simulink model "TiltCopter_Simulator"  (R2015a)
settings: Solver=ode45  StartTime=0.0  StopTime=10.0  RelTol=1e-3
values from neighbouring files (symbols this model uses):
  b = 0.55/2    (= 0.275)    [TiltCopter_Parameters.m]
  B0 = 1.399e04    (= 13990)    [TiltCopter_Parameters.m]
  B1 = 1150    [TiltCopter_Parameters.m]
  B2 = 37.46    [TiltCopter_Parameters.m]
  B3 = 1    [TiltCopter_Parameters.m]
  dLMN = [dLdp  0    0 ... (first row only)    [TiltCopter_Parameters.m]
  Fx = 0.5    [Main_tiltCopter.m]
  Fy = 0    [Main_tiltCopter.m]
  g = 9.81    [TiltCopter_Parameters.m]
  In = diag([Ixx Iyy Izz])    [TiltCopter_Parameters.m]
  InInv = In\eye(3)    [TiltCopter_Parameters.m]
  Kq = Cq*ro*A*R^3    (= 2.88925724261e-07)    [TiltCopter_Parameters.m]
  Kt = Ct*ro*A*R^2    (= 2.46191978476e-05)    [TiltCopter_Parameters.m]
  L = 0    [Main_tiltCopter.m]
  M = 0    [Main_tiltCopter.m]
  m = 1.478    [TiltCopter_Parameters.m]
  m_servo = p(1)    [TiltCopter_Parameters.m]
  Mb = diag([m m m])    [TiltCopter_Parameters.m]
  MbInv = Mb\eye(3)    [TiltCopter_Parameters.m]
  N = 0    [Main_tiltCopter.m]
  omega_hover = OMEhov    [TiltCopter_Parameters.m]
  q_servo = p(2)    [TiltCopter_Parameters.m]
  ServoMotor_Gain = 1.409e04    (= 14090)    [TiltCopter_Parameters.m]
  T = -20    [Main_tiltCopter.m]
  tau = 0.055257    [TiltCopter_Parameters.m]
  x1 = [m q]    [TiltCopter_Parameters.m]
libraries: aerolibutil x2
settings Model: Creator=Claudio  LastModifiedBy=Claudio

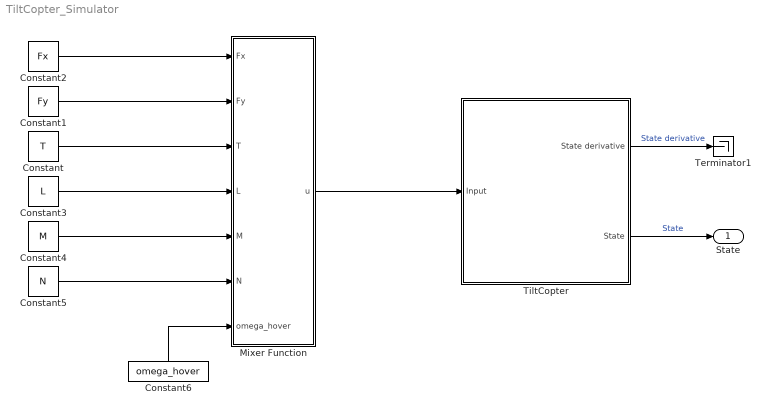
== system TiltCopter_Simulator ==
  Constant : Constant  Value=T
  Constant1 : Constant  Value=Fy
  Constant2 : Constant  Value=Fx
  Constant3 : Constant  Value=L
  Constant4 : Constant  Value=M
  Constant5 : Constant  Value=N
  Constant6 : Constant  Value=omega_hover
  Mixer Function : Subsystem
  Terminator1 : Terminator
  TiltCopter : Subsystem
      mask Display:
      | % image(imread(''))
      | port_label('input',1,'u')
      | port_label('output',1,'Xdot')
      | port_label('output',2,'X')
  State : Outport
  wires:
  TiltCopter/2(State) -> State/1  "State"
  TiltCopter/1(State derivative) -> Terminator1/1  "State derivative"
  Constant2/1 -> Mixer Function/1(Fx)
  Constant1/1 -> Mixer Function/2(Fy)
  Constant/1 -> Mixer Function/3(T)
  Constant3/1 -> Mixer Function/4(L)
  Constant4/1 -> Mixer Function/5(M)
  Constant5/1 -> Mixer Function/6(N)
  Constant6/1 -> Mixer Function/7(omega_hover)
  Mixer Function/1(u) -> TiltCopter/1(Input)

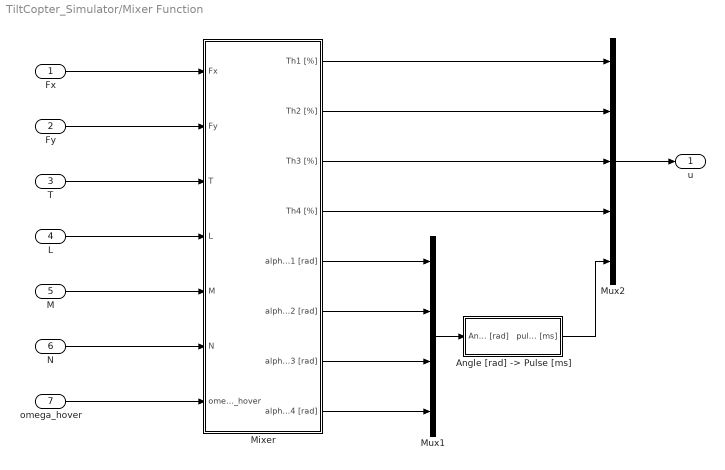
== system TiltCopter_Simulator/Mixer Function ==
  Fx : Inport
  Fy : Inport  Port=2
  T : Inport  Port=3
  L : Inport  Port=4
  M : Inport  Port=5
  N : Inport  Port=6
  omega_hover : Inport  Port=7
  "Angle [rad] -> Pulse [ms]" : Subsystem
  Mixer : Subsystem
  Mux1 : Mux
  Mux2 : Mux  Inputs=5
  u : Outport
  wires:
  Mux2/1 -> u/1
  Fy/1 -> Mixer/2(Fy)
  Fx/1 -> Mixer/1(Fx)
  T/1 -> Mixer/3(T)
  L/1 -> Mixer/4(L)
  N/1 -> Mixer/6(N)
  omega_hover/1 -> Mixer/7(omega_hover)
  M/1 -> Mixer/5(M)
  Mixer/7(alpha_3 [rad]) -> Mux1/3
  Mixer/2(Th2 [%]) -> Mux2/2
  Mixer/3(Th3 [%]) -> Mux2/3
  Mixer/4(Th4 [%]) -> Mux2/4
  Mixer/5(alpha_1 [rad]) -> Mux1/1
  Mixer/6(alpha_2 [rad]) -> Mux1/2
  Mixer/8(alpha_4 [rad]) -> Mux1/4
  "Angle [rad] -> Pulse [ms]"/1(pulse [ms]) -> Mux2/5
  Mux1/1 -> "Angle [rad] -> Pulse [ms]"/1(Angle [rad])
  Mixer/1(Th1 [%]) -> Mux2/1

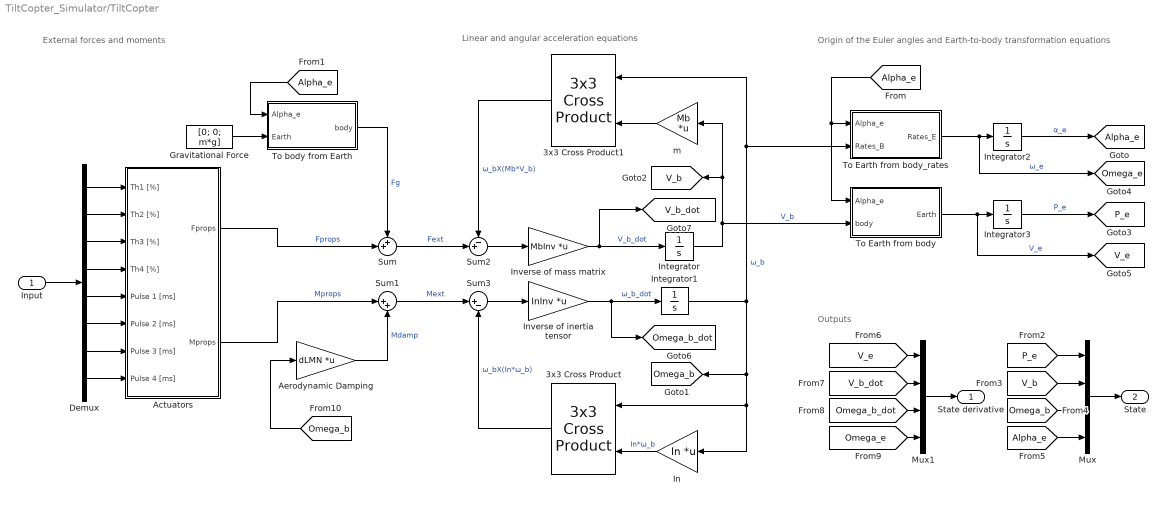
== system TiltCopter_Simulator/TiltCopter ==
  note: External forces and moments
  note: Outputs
  note: Origin of the Euler angles and Earth-to-body transformation equations
  note: Linear and angular acceleration equations
  Input : Inport
  3x3 Cross Product : aerolibutil/3x3 Cross Product
  3x3 Cross Product1 : aerolibutil/3x3 Cross Product
  Actuators : Subsystem
  Aerodynamic Damping : Gain  Gain=dLMN  Multiplication=Matrix(K*u)
  Demux : Demux  Outputs=8
  Gravitational Force : Constant  Value=[0; 0; m*g]
  In : Gain  Gain=In  Multiplication=Matrix(K*u)
  Integrator{,1..3} (4 alike) : Integrator  InitialCondition=[0; 0; 0]
  Inverse of inertia tensor : Gain  Gain=InInv  Multiplication=Matrix(K*u)
  Inverse of mass matrix : Gain  Gain=MbInv  Multiplication=Matrix(K*u)
  Mux : Mux
  Mux1 : Mux
  Sum : Sum  Inputs=++|
  Sum1 : Sum  Inputs=|++
  Sum2 : Sum  Inputs=-+|
  Sum3 : Sum  Inputs=|+-
  To Earth from body : MATLAB Function  TreatAsAtomicUnit=on
  To Earth from body_rates : MATLAB Function  TreatAsAtomicUnit=on
  To body from Earth : MATLAB Function  TreatAsAtomicUnit=on
  m : Gain  Gain=Mb  Multiplication=Matrix(K*u)
  State derivative : Outport
  State : Outport  Port=2
  tag scope: Alpha_e=global, Omega_b=global, Omega_b_dot=global, Omega_e=global, P_e=global, V_b=global, V_b_dot=global, V_e=global
  wires:
  To Earth from body_rates/1(Rates_E) -> Integrator2/1, [Omega_e]  "ω_e"
  [P_e] -> Mux/1
  Actuators/2(Mprops) -> Sum1/1  "Mprops"
  3x3 Cross Product/1 -> Sum3/2  "ω_bX(In*ω_b)"
  [V_b_dot] -> Mux1/2
  Mux/1 -> State/1
  Mux1/1 -> State derivative/1
  [V_b] -> Mux/2
  [Alpha_e] -> Mux/4
  [Omega_b] -> Mux/3
  Demux/4 -> Actuators/4(Th4 [%])
  [Omega_e] -> Mux1/4
  [Omega_b_dot] -> Mux1/3
  [V_e] -> Mux1/1
  Demux/3 -> Actuators/3(Th3 [%])
  Inverse of mass matrix/1 -> Integrator/1, [V_b_dot]  "V_b_dot"
  Integrator/1 -> To Earth from body/2(body), m/1, [V_b]  "V_b"
  [Alpha_e] -> To Earth from body/1(Alpha_e), To Earth from body_rates/1(Alpha_e)
  Integrator1/1 -> To Earth from body_rates/2(Rates_B), 3x3 Cross Product1/1, 3x3 Cross Product/1, In/1, [Omega_b]  "ω_b"
  Sum3/1 -> Inverse of inertia tensor/1
  Sum2/1 -> Inverse of mass matrix/1
  m/1 -> 3x3 Cross Product1/2
  Sum/1 -> Sum2/2  "Fext"
  Sum1/1 -> Sum3/1  "Mext"
  Demux/1 -> Actuators/1(Th1 [%])
  Demux/2 -> Actuators/2(Th2 [%])
  Inverse of inertia tensor/1 -> Integrator1/1, [Omega_b_dot]  "ω_b_dot"
  3x3 Cross Product1/1 -> Sum2/1  "ω_bX(Mb*V_b)"
  Integrator2/1 -> [Alpha_e]  "α_e"
  Aerodynamic Damping/1 -> Sum1/2  "Mdamp"
  Actuators/1(Fprops) -> Sum/2  "Fprops"
  Integrator3/1 -> [P_e]  "P_e"
  In/1 -> 3x3 Cross Product/2  "In*ω_b"
  [Omega_b] -> Aerodynamic Damping/1
  To Earth from body/1(Earth) -> [V_e], Integrator3/1  "V_e"
  To body from Earth/1(body) -> Sum/1  "Fg"
  Gravitational Force/1 -> To body from Earth/2(Earth)
  [Alpha_e] -> To body from Earth/1(Alpha_e)
  Input/1 -> Demux/1
  Demux/5 -> Actuators/5(Pulse 1 [ms])
  Demux/6 -> Actuators/6(Pulse 2 [ms])
  Demux/7 -> Actuators/7(Pulse 3 [ms])
  Demux/8 -> Actuators/8(Pulse 4 [ms])

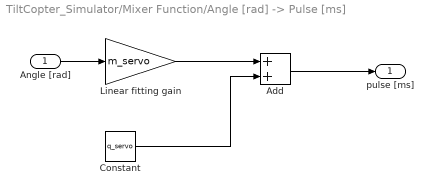
== system TiltCopter_Simulator/Mixer Function/Angle [rad] -> Pulse [ms] ==
  Angle [rad] : Inport
  Add : Sum
  Constant : Constant  Value=q_servo
  Linear fitting gain : Gain  Gain=m_servo
  pulse [ms] : Outport
  wires:
  Angle [rad]/1 -> Linear fitting gain/1
  Constant/1 -> Add/2
  Linear fitting gain/1 -> Add/1
  Add/1 -> pulse [ms]/1

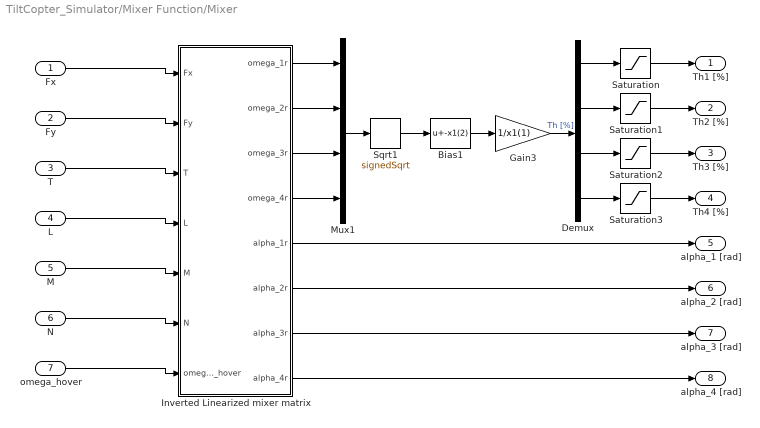
== system TiltCopter_Simulator/Mixer Function/Mixer ==
  Fx : Inport
  Fy : Inport  Port=2
  T : Inport  Port=3
  L : Inport  Port=4
  M : Inport  Port=5
  N : Inport  Port=6
  omega_hover : Inport  Port=7
  Bias1 : Bias  Bias=-x1(2)
  Demux : Demux
  Gain3 : Gain  Gain=1/x1(1)
  Inverted Linearized mixer matrix : MATLAB Function  TreatAsAtomicUnit=on
  Mux1 : Mux
  Saturation{,1..3} (4 alike) : Saturate  UpperLimit=100  LowerLimit=0
  Sqrt1 : Sqrt  Operator=signedSqrt  SaturateOnIntegerOverflow=on
  Th1 [%] : Outport
  Th2 [%] : Outport  Port=2
  Th3 [%] : Outport  Port=3
  Th4 [%] : Outport  Port=4
  alpha_1 [rad] : Outport  Port=5
  alpha_2 [rad] : Outport  Port=6
  alpha_3 [rad] : Outport  Port=7
  alpha_4 [rad] : Outport  Port=8
  wires:
  T/1 -> Inverted Linearized mixer matrix/3(T)
  Inverted Linearized mixer matrix/4(omega_4r) -> Mux1/4
  Fx/1 -> Inverted Linearized mixer matrix/1(Fx)
  N/1 -> Inverted Linearized mixer matrix/6(N)
  Inverted Linearized mixer matrix/2(omega_2r) -> Mux1/2
  Inverted Linearized mixer matrix/1(omega_1r) -> Mux1/1
  omega_hover/1 -> Inverted Linearized mixer matrix/7(omega_hover)
  Inverted Linearized mixer matrix/3(omega_3r) -> Mux1/3
  M/1 -> Inverted Linearized mixer matrix/5(M)
  Fy/1 -> Inverted Linearized mixer matrix/2(Fy)
  L/1 -> Inverted Linearized mixer matrix/4(L)
  Inverted Linearized mixer matrix/7(alpha_3r) -> alpha_3 [rad]/1
  Demux/1 -> Saturation/1
  Saturation/1 -> Th1 [%]/1
  Demux/2 -> Saturation1/1
  Demux/3 -> Saturation2/1
  Demux/4 -> Saturation3/1
  Saturation3/1 -> Th4 [%]/1
  Saturation2/1 -> Th3 [%]/1
  Saturation1/1 -> Th2 [%]/1
  Gain3/1 -> Demux/1  "Th [%]"
  Inverted Linearized mixer matrix/5(alpha_1r) -> alpha_1 [rad]/1
  Inverted Linearized mixer matrix/8(alpha_4r) -> alpha_4 [rad]/1
  Bias1/1 -> Gain3/1
  Mux1/1 -> Sqrt1/1
  Sqrt1/1 -> Bias1/1
  Inverted Linearized mixer matrix/6(alpha_2r) -> alpha_2 [rad]/1

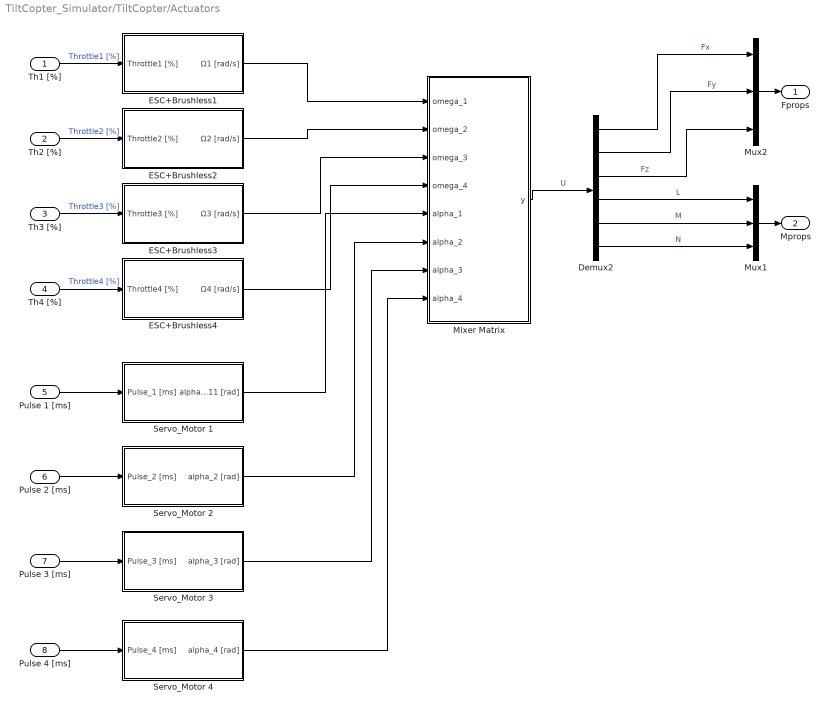
== system TiltCopter_Simulator/TiltCopter/Actuators ==
  Th1 [%] : Inport
  Th2 [%] : Inport  Port=2
  Th3 [%] : Inport  Port=3
  Th4 [%] : Inport  Port=4
  Pulse 1 [ms] : Inport  Port=5
  Pulse 2 [ms] : Inport  Port=6
  Pulse 3 [ms] : Inport  Port=7
  Pulse 4 [ms] : Inport  Port=8
  Demux2 : Demux  Outputs=6
  ESC+Brushless1 : Subsystem
  ESC+Brushless2 : Subsystem
  ESC+Brushless3 : Subsystem
  ESC+Brushless4 : Subsystem
  Mixer Matrix : MATLAB Function  TreatAsAtomicUnit=on
  Mux1 : Mux  Inputs=3
  Mux2 : Mux  Inputs=3
  Servo_Motor 1 : Subsystem
  Servo_Motor 2 : Subsystem
  Servo_Motor 3 : Subsystem
  Servo_Motor 4 : Subsystem
  Fprops : Outport
  Mprops : Outport  Port=2
  wires:
  Mixer Matrix/1(y) -> Demux2/1  "U"
  Th1 [%]/1 -> ESC+Brushless1/1(Throttle1 [%])  "Throttle1 [%]"
  Th2 [%]/1 -> ESC+Brushless2/1(Throttle2 [%])  "Throttle2 [%]"
  Th4 [%]/1 -> ESC+Brushless4/1(Throttle4 [%])  "Throttle4 [%]"
  Th3 [%]/1 -> ESC+Brushless3/1(Throttle3 [%])  "Throttle3 [%]"
  Mux1/1 -> Mprops/1
  Mux2/1 -> Fprops/1
  Pulse 1 [ms]/1 -> Servo_Motor 1/1(Pulse_1 [ms])
  Pulse 2 [ms]/1 -> Servo_Motor 2/1(Pulse_2 [ms])
  Pulse 3 [ms]/1 -> Servo_Motor 3/1(Pulse_3 [ms])
  Pulse 4 [ms]/1 -> Servo_Motor 4/1(Pulse_4 [ms])
  ESC+Brushless1/1(Ω1 [rad/s]) -> Mixer Matrix/1(omega_1)
  ESC+Brushless2/1(Ω2 [rad/s]) -> Mixer Matrix/2(omega_2)
  ESC+Brushless3/1(Ω3 [rad/s]) -> Mixer Matrix/3(omega_3)
  ESC+Brushless4/1(Ω4 [rad/s]) -> Mixer Matrix/4(omega_4)
  Servo_Motor 2/1(alpha_2 [rad]) -> Mixer Matrix/6(alpha_2)
  Servo_Motor 3/1(alpha_3 [rad]) -> Mixer Matrix/7(alpha_3)
  Servo_Motor 4/1(alpha_4 [rad]) -> Mixer Matrix/8(alpha_4)
  Demux2/1 -> Mux2/1  "Fx"
  Demux2/2 -> Mux2/2  "Fy"
  Demux2/3 -> Mux2/3  "Fz"
  Demux2/4 -> Mux1/1  "L"
  Demux2/5 -> Mux1/2  "M"
  Demux2/6 -> Mux1/3  "N"
  Servo_Motor 1/1(alpha_11 [rad]) -> Mixer Matrix/5(alpha_1)

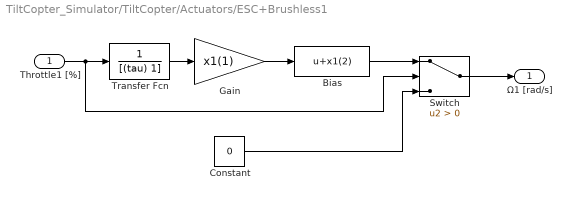
== system TiltCopter_Simulator/TiltCopter/Actuators/ESC+Brushless1 ==
  Throttle1 [%] : Inport
  Bias : Bias  Bias=x1(2)
  Constant : Constant  Value=0
  Gain : Gain  Gain=x1(1)
  Switch : Switch  Criteria=u2 > Threshold
  Transfer Fcn : TransferFcn  Denominator=[(tau) 1]
  Ω1 [rad/s] : Outport
  wires:
  Gain/1 -> Bias/1
  Bias/1 -> Switch/1
  Constant/1 -> Switch/3
  Switch/1 -> Ω1 [rad/s]/1
  Throttle1 [%]/1 -> Transfer Fcn/1, Switch/2
  Transfer Fcn/1 -> Gain/1

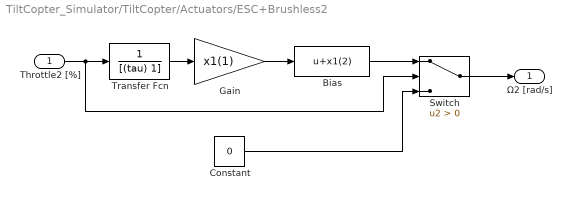
== system TiltCopter_Simulator/TiltCopter/Actuators/ESC+Brushless2 ==
  Throttle2 [%] : Inport
  Bias : Bias  Bias=x1(2)
  Constant : Constant  Value=0
  Gain : Gain  Gain=x1(1)
  Switch : Switch  Criteria=u2 > Threshold
  Transfer Fcn : TransferFcn  Denominator=[(tau) 1]
  Ω2 [rad/s] : Outport
  wires:
  Switch/1 -> Ω2 [rad/s]/1
  Constant/1 -> Switch/3
  Bias/1 -> Switch/1
  Gain/1 -> Bias/1
  Throttle2 [%]/1 -> Transfer Fcn/1, Switch/2
  Transfer Fcn/1 -> Gain/1

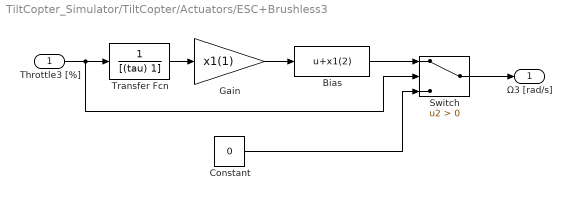
== system TiltCopter_Simulator/TiltCopter/Actuators/ESC+Brushless3 ==
  Throttle3 [%] : Inport
  Bias : Bias  Bias=x1(2)
  Constant : Constant  Value=0
  Gain : Gain  Gain=x1(1)
  Switch : Switch  Criteria=u2 > Threshold
  Transfer Fcn : TransferFcn  Denominator=[(tau) 1]
  Ω3 [rad/s] : Outport
  wires:
  Gain/1 -> Bias/1
  Bias/1 -> Switch/1
  Constant/1 -> Switch/3
  Switch/1 -> Ω3 [rad/s]/1
  Throttle3 [%]/1 -> Transfer Fcn/1, Switch/2
  Transfer Fcn/1 -> Gain/1

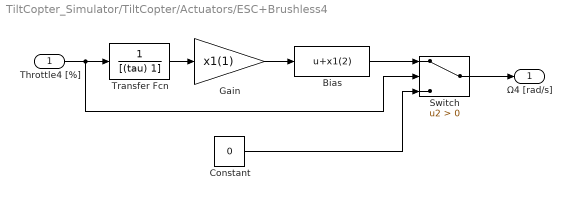
== system TiltCopter_Simulator/TiltCopter/Actuators/ESC+Brushless4 ==
  Throttle4 [%] : Inport
  Bias : Bias  Bias=x1(2)
  Constant : Constant  Value=0
  Gain : Gain  Gain=x1(1)
  Switch : Switch  Criteria=u2 > Threshold
  Transfer Fcn : TransferFcn  Denominator=[(tau) 1]
  Ω4 [rad/s] : Outport
  wires:
  Switch/1 -> Ω4 [rad/s]/1
  Constant/1 -> Switch/3
  Bias/1 -> Switch/1
  Gain/1 -> Bias/1
  Throttle4 [%]/1 -> Transfer Fcn/1, Switch/2
  Transfer Fcn/1 -> Gain/1

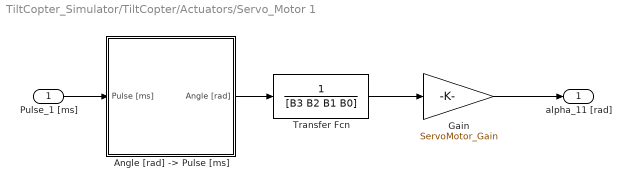
== system TiltCopter_Simulator/TiltCopter/Actuators/Servo_Motor 1 ==
  Pulse_1 [ms] : Inport
  "Angle [rad] -> Pulse [ms]" : Subsystem
  Gain : Gain  Gain=ServoMotor_Gain
  Transfer Fcn : TransferFcn  Denominator=[B3 B2 B1 B0]
  alpha_11 [rad] : Outport
  wires:
  Gain/1 -> alpha_11 [rad]/1
  Transfer Fcn/1 -> Gain/1
  "Angle [rad] -> Pulse [ms]"/1(Angle [rad]) -> Transfer Fcn/1
  Pulse_1 [ms]/1 -> "Angle [rad] -> Pulse [ms]"/1(Pulse [ms])

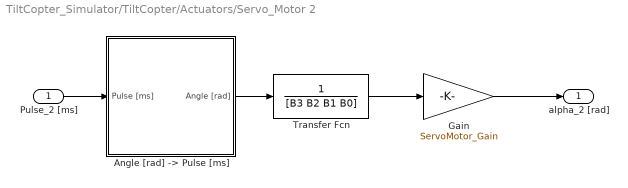
== system TiltCopter_Simulator/TiltCopter/Actuators/Servo_Motor 2 ==
  Pulse_2 [ms] : Inport
  "Angle [rad] -> Pulse [ms]" : Subsystem
  Gain : Gain  Gain=ServoMotor_Gain
  Transfer Fcn : TransferFcn  Denominator=[B3 B2 B1 B0]
  alpha_2 [rad] : Outport
  wires:
  Gain/1 -> alpha_2 [rad]/1
  Transfer Fcn/1 -> Gain/1
  "Angle [rad] -> Pulse [ms]"/1(Angle [rad]) -> Transfer Fcn/1
  Pulse_2 [ms]/1 -> "Angle [rad] -> Pulse [ms]"/1(Pulse [ms])

== system TiltCopter_Simulator/TiltCopter/Actuators/Servo_Motor 3 ==
  Pulse_3 [ms] : Inport
  "Angle [rad] -> Pulse [ms]" : Subsystem
  Gain : Gain  Gain=ServoMotor_Gain
  Transfer Fcn : TransferFcn  Denominator=[B3 B2 B1 B0]
  alpha_3 [rad] : Outport
  wires:
  Gain/1 -> alpha_3 [rad]/1
  Transfer Fcn/1 -> Gain/1
  "Angle [rad] -> Pulse [ms]"/1(Angle [rad]) -> Transfer Fcn/1
  Pulse_3 [ms]/1 -> "Angle [rad] -> Pulse [ms]"/1(Pulse [ms])

== system TiltCopter_Simulator/TiltCopter/Actuators/Servo_Motor 4 ==
  Pulse_4 [ms] : Inport
  "Angle [rad] -> Pulse [ms]" : Subsystem
  Gain : Gain  Gain=ServoMotor_Gain
  Transfer Fcn : TransferFcn  Denominator=[B3 B2 B1 B0]
  alpha_4 [rad] : Outport
  wires:
  Gain/1 -> alpha_4 [rad]/1
  Transfer Fcn/1 -> Gain/1
  "Angle [rad] -> Pulse [ms]"/1(Angle [rad]) -> Transfer Fcn/1
  Pulse_4 [ms]/1 -> "Angle [rad] -> Pulse [ms]"/1(Pulse [ms])

== system TiltCopter_Simulator/TiltCopter/Actuators/Servo_Motor 1/Angle [rad] -> Pulse [ms] ==
  Pulse [ms] : Inport
  Add : Sum  Inputs=+-
  Constant : Constant  Value=q_servo
  Linear fitting gain : Gain  Gain=1/m_servo
  Angle [rad] : Outport
  wires:
  Constant/1 -> Add/2
  Add/1 -> Linear fitting gain/1
  Pulse [ms]/1 -> Add/1
  Linear fitting gain/1 -> Angle [rad]/1

== system TiltCopter_Simulator/TiltCopter/Actuators/Servo_Motor 2/Angle [rad] -> Pulse [ms] ==
  Pulse [ms] : Inport
  Add : Sum  Inputs=+-
  Constant : Constant  Value=q_servo
  Linear fitting gain : Gain  Gain=1/m_servo
  Angle [rad] : Outport
  wires:
  Constant/1 -> Add/2
  Add/1 -> Linear fitting gain/1
  Pulse [ms]/1 -> Add/1
  Linear fitting gain/1 -> Angle [rad]/1

== system TiltCopter_Simulator/TiltCopter/Actuators/Servo_Motor 3/Angle [rad] -> Pulse [ms] ==
  Pulse [ms] : Inport
  Add : Sum  Inputs=+-
  Constant : Constant  Value=q_servo
  Linear fitting gain : Gain  Gain=1/m_servo
  Angle [rad] : Outport
  wires:
  Constant/1 -> Add/2
  Add/1 -> Linear fitting gain/1
  Pulse [ms]/1 -> Add/1
  Linear fitting gain/1 -> Angle [rad]/1

== system TiltCopter_Simulator/TiltCopter/Actuators/Servo_Motor 4/Angle [rad] -> Pulse [ms] ==
  Pulse [ms] : Inport
  Add : Sum  Inputs=+-
  Constant : Constant  Value=q_servo
  Linear fitting gain : Gain  Gain=1/m_servo
  Angle [rad] : Outport
  wires:
  Constant/1 -> Add/2
  Add/1 -> Linear fitting gain/1
  Pulse [ms]/1 -> Add/1
  Linear fitting gain/1 -> Angle [rad]/1

== matlab function TiltCopter_Simulator/TiltCopter/To body from Earth ==
  data: Alpha_e input; Earth input; body output
 function body = Tbe(Alpha_e, Earth)
%#codegen
phi = Alpha_e(1);
theta = Alpha_e(2);
psi = Alpha_e(3);

Sphi = sin(phi);
Cphi = cos(phi);
Stheta = sin(theta);
Ctheta = cos(theta);
Spsi = sin(psi);
Cpsi = cos(psi);

TBE = [        Ctheta*Cpsi               Ctheta*Spsi          -Stheta    ;
       Sphi*Stheta*Cpsi-Cphi*Spsi Sphi*Stheta*Spsi+Cphi*Cpsi Sphi*Ctheta ;
       Cphi*Stheta*Cpsi+Sphi*Spsi Cphi*Stheta*Spsi-Sphi*Cpsi Cphi*Ctheta];

body = TBE* Earth;

== matlab function TiltCopter_Simulator/TiltCopter/To Earth from body ==
  data: Alpha_e input; Earth output; body input
 function Earth = Tbet(Alpha_e, body)
%#codegen
phi = Alpha_e(1);
theta = Alpha_e(2);
psi = Alpha_e(3);

Sphi = sin(phi);
Cphi = cos(phi);
Stheta = sin(theta);
Ctheta = cos(theta);
Spsi = sin(psi);
Cpsi = cos(psi);

TBE = [        Ctheta*Cpsi               Ctheta*Spsi          -Stheta    ;
       Sphi*Stheta*Cpsi-Cphi*Spsi Sphi*Stheta*Spsi+Cphi*Cpsi Sphi*Ctheta ;
       Cphi*Stheta*Cpsi+Sphi*Spsi Cphi*Stheta*Spsi-Sphi*Cpsi Cphi*Ctheta];
TEB = TBE';

Earth = TEB* body;

== matlab function TiltCopter_Simulator/TiltCopter/To Earth from body_rates ==
  data: Alpha_e input; Rates_B input; Rates_E output
 function Rates_E = Einv(Alpha_e, Rates_B)
%#codegen
phi = Alpha_e(1);
theta = Alpha_e(2);

Sphi = sin(phi);
Cphi = cos(phi);
Ctheta = cos(theta);
Ttheta = tan(theta);

Einv = [1   Sphi*Ttheta    Cphi*Ttheta ;
        0       Cphi          -Sphi    ;
        0   Sphi/Ctheta    Cphi/Ctheta];

Rates_E = Einv* Rates_B;

== matlab function TiltCopter_Simulator/TiltCopter/Actuators/Mixer Matrix ==
  data: omega_1 input; y output; omega_2 input; omega_3 input; omega_4 input; alpha_1 input; alpha_2 input; alpha_3 input; alpha_4 input; Kt parameter; Kq parameter; b parameter
function y = fcn(omega_1,omega_2,omega_3,omega_4,alpha_1,alpha_2,alpha_3,alpha_4,Kt,Kq,b)
%#codegen


% F_ext comumns are [Fx;Fy;Fz]
F_ext =[ Kt*sin(alpha_2)*omega_2^2 - Kt*sin(alpha_4)*omega_4^2;
         - Kt*sin(alpha_1)*omega_1^2 + Kt*sin(alpha_3)*omega_3^2;
         - Kt*cos(alpha_1)*omega_1^2 - Kt*cos(alpha_2)*omega_2^2 - Kt*cos(alpha_3)*omega_3^2 - Kt*cos(alpha_4)*omega_4^2 
        ];

% M_ext colums are [M_roll;M_Pitch;M_yaw]    
M_ext =[ Kq*omega_2^2*sin(alpha_2) - Kq*omega_4^2*sin(alpha_4) - Kt*b*omega_2^2*cos(alpha_2) + Kt*b*omega_4^2*cos(alpha_4);
         Kq*omega_1^2*sin(alpha_1) - Kq*omega_3^2*sin(alpha_3) + Kt*b*omega_1^2*cos(alpha_1) - Kt*b*omega_3^2*cos(alpha_3);
         Kq*omega_1^2*cos(alpha_1) - Kq*omega_2^2*cos(alpha_2) + Kq*omega_3^2*cos(alpha_3) - Kq*omega_4^2*cos(alpha_4) - Kt*b*omega_1^2*sin(alpha_1) - Kt*b*omega_2^2*sin(alpha_2) - Kt*b*omega_3^2*sin(alpha_3) - Kt*b*omega_4^2*sin(alpha_4);
       ];
 

y = [F_ext;M_ext];

== matlab function TiltCopter_Simulator/Mixer Function/Mixer/Inverted Linearized mixer matrix ==
  data: Fx input; Fy input; T input; L input; M input; N input; omega_1r output; omega_hover input; Kt parameter; Kq parameter; b parameter; omega_2r output; omega_3r output; omega_4r output; alpha_1r output; alpha_2r output; alpha_3r output; alpha_4r output
function [omega_1r,omega_2r,omega_3r,omega_4r,alpha_1r,alpha_2r,alpha_3r,alpha_4r] = fcn(Fx,Fy,T,L,M,N,omega_hover,Kt,Kq,b)
%#codegen

omega_1 = omega_hover;
omega_2 = omega_hover;
omega_3 = omega_hover;
omega_4 = omega_hover;

% Calcolo prima gli alpha per ottenere la Fx e Fy desiderata considerando
% una omega di hovering
alpha_2 = -asin(Fx/(Kt*(omega_2^2 + omega_4^2)));

alpha_1 = asin(Fy/(Kt*(omega_1^2 + omega_3^2)));
alpha_3 = -alpha_1;
alpha_4 = -alpha_2;

% A questo punto risolvo la matrice K_mix, considerando gli angoli noti e
% risolvo solo per omega_i
K_mix = [
    -Kt*cos(alpha_1),                      -Kt*cos(alpha_2),                    -Kt*cos(alpha_3),                    -Kt*cos(alpha_4);
                                   0, - Kq*sin(alpha_2) - Kt*b*cos(alpha_2),                                   0, Kq*sin(alpha_4) + Kt*b*cos(alpha_4);
 Kt*b*cos(alpha_1) - Kq*sin(alpha_1),                                     0, Kq*sin(alpha_3) - Kt*b*cos(alpha_3),                                   0;
 Kq*cos(alpha_1) + Kt*b*sin(alpha_1),   Kt*b*sin(alpha_2) - Kq*cos(alpha_2), Kq*cos(alpha_3) + Kt*b*sin(alpha_3), Kt*b*sin(alpha_4) - Kq*cos(alpha_4)]

Omega_result = inv(K_mix)*[T;L;M;N];
%y = [Omega_result;alpha_1;alpha_2];
omega_1r = Omega_result(1);
omega_2r = Omega_result(2);
omega_3r = Omega_result(3);
omega_4r = Omega_result(4);
alpha_1r = alpha_1;
alpha_2r = alpha_2;
alpha_3r = -alpha_1;
alpha_4r = -alpha_2;
